simulink model "et_robocon_dev_guy3"  (R2013b)
settings: Solver=FixedStepDiscrete  SolverMode=SingleTasking  StartTime=0.0  StopTime=inf  FixedStep=balancer_ts  RelTol=1e-3
undefined symbols (not defined in the file): a_d, a_r, balancerStates_Bus0, Batt, battery_gain, battery_offset, cmd_max, current_mode_status, current_task_operation_status, DiscIntNeverNeededParam, exec_period, gcbh, Init_Bus0, K, k_f, k_i, k_phidot, k_thetadot, lightCalib, R, realtime, STATE, TRACK_MODE_LIST, ts2, W
libraries: legonxtlib x34, simulink x11, simulink_extras x4
(part 1 of 4)
settings Model: DataDictionary=mainDict.sldd  ExtModeTrigDuration=2  Creator=mbiesiad  LastModifiedBy=grouleau
settings ConfigSet: Description=Use this configuration to communicate between two robots. This robot is the master.
settings OptimizationCC: OptimizeModelRefInitCode=on  LifeSpan=1
settings DebuggingCC: UnderspecifiedInitializationDetection=Simplified  SolverPrmCheckMsg=none  ParameterPrecisionLossMsg=none  SignalLabelMismatchMsg=error  NonBusSignalsTreatedAsBus=error
settings HardwareCC: ProdLargestAtomicInteger=Long  ProdLargestAtomicFloat=Float  ProdEndianess=LittleEndian  ProdHWDeviceType=ARM Compatible->ARM 7
settings RTWCC: SystemTargetFile=realtime.tlc  GenerateMakefile=off  TemplateMakefile=realtime.tmf  Description=Run on Target Hardware  RTWVerbose=off  ProcessScript=realtime_make_rtw_hook
settings STFCustomTargetCC: TargetLibSuffix=.a  GenerateSampleERTMain=on  ERTCustomFileBanners=on  SupportNonInlinedSFcns=off  SupportVariableSizeSignals=on  MATLABClassNameForMDSCustomization=Simulink.SoftwareTarget.ERTCustomization  GRTInterface=off  SystemTargetFile=realtime.tlc
settings ERTTargetCC: CodeReplacementLibrary=ANSI_C  GenerateSampleERTMain=on  ParMdlRefBuildCompliant=off  CompOptLevelCompliant=off  ConcurrentExecutionCompliant=off  CombineOutputUpdateFcns=off  ERTFirstTimeCompliant=off  SupportContinuousTime=on  SupportVariableSizeSignals=on  ModelStepFunctionPrototypeControlCompliant=off  CPPClassGenCompliant=off  ExtModeTransport=1  ExtModeMexFile=ext_serial_win32_comm_no_acks_rtt_byteswap  ExtModeMexArgs=0 1 9600  InlinedParameterPlacement=NonHierarchical  ERTSrcFileBannerTemplate=realtime_code_template.cgt  ERTHdrFileBannerTemplate=realtime_code_template.cgt  ERTDataSrcFileTemplate=realtime_code_template.cgt  ERTDataHdrFileTemplate=realtime_code_template.cgt  ERTCustomFileTemplate=realtime_file_process.tlc

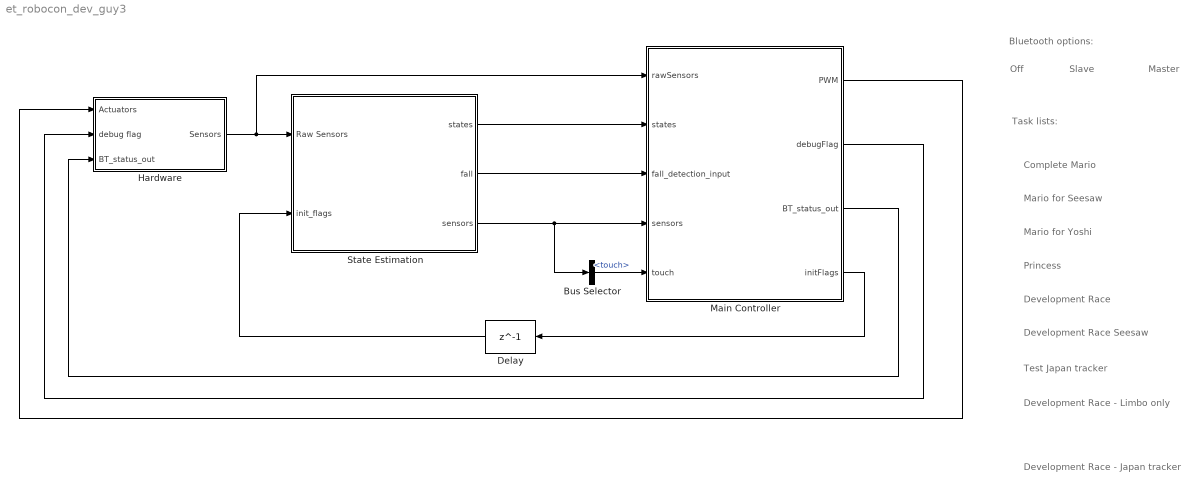
== system et_robocon_dev_guy3 ==
  note: Task lists:
  note: Bluetooth options:
  note: Slave
  note: Complete Mario
  note: Princess
  note: Mario for Seesaw
  note: Mario for Yoshi
  note: Development Race
  note: Development Race Seesaw
  note: Master
  note: Off
  note: Development Race - Japan tracker
  note: Test Japan tracker
  note: Development Race - Limbo only
  Bus Selector : BusSelector  OutputSignals=touch
  Delay : Delay  DelayLength=1
  Hardware : Subsystem  VariantControl=Variant1
  Main Controller : Stateflow chart  TreatAsAtomicUnit=on
  State Estimation : Subsystem
  wires:
  State Estimation/2(fall) -> Main Controller/3(fall_detection_input)
  State Estimation/3(sensors) -> Bus Selector/1, Main Controller/4(sensors)
  Bus Selector/1 -> Main Controller/5(touch)  "<touch>"
  Hardware/1(Sensors) -> Main Controller/1(rawSensors), State Estimation/1(Raw Sensors)
  Main Controller/4(initFlags) -> Delay/1
  State Estimation/1(states) -> Main Controller/2(states)
  Delay/1 -> State Estimation/2(init_flags)
  Main Controller/2(debugFlag) -> Hardware/2(debug flag)
  Main Controller/1(PWM) -> Hardware/1(Actuators)
  Main Controller/3(BT_status_out) -> Hardware/3(BT_status_out)

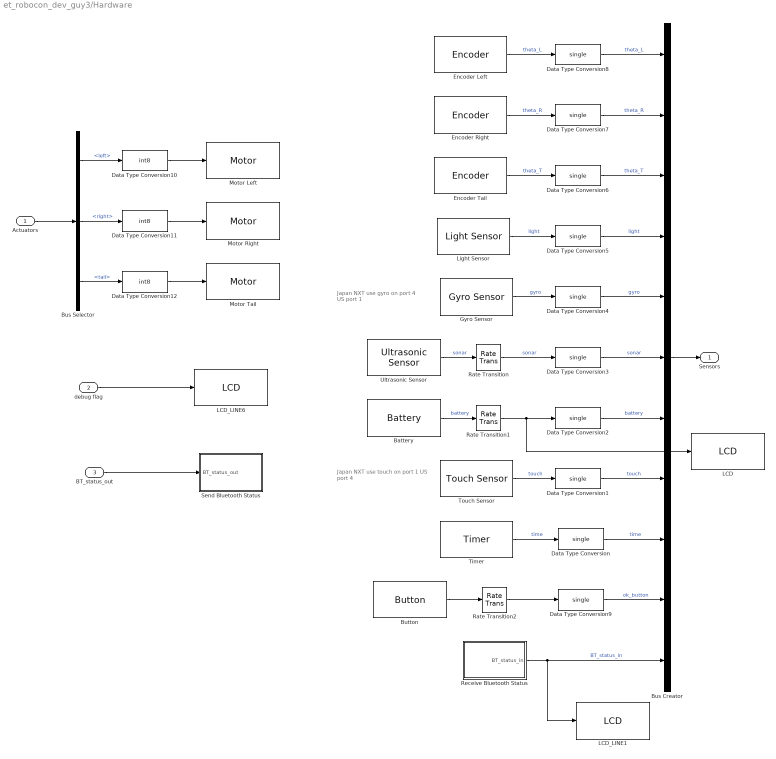
== system et_robocon_dev_guy3/Hardware ==
  note: Japan NXT use gyro on port 4
      | US port 1
  note: Japan NXT use touch  on port 1
      | US port 4
  Actuators : Inport
  debug flag : Inport  Port=2
  BT_status_out : Inport  Port=3
  Battery : legonxtlib/Battery  sampleTime=.1
  Bus Creator : BusCreator  Inputs=11
  Bus Selector : BusSelector  OutputSignals=left,right,tail
  Button : legonxtlib/Button  buttonType=Middle orange  sampleTime=0.1
  Data Type Conversion{,1..9} (10 alike) : DataTypeConversion  OutDataTypeStr=single
  Data Type Conversion10 : DataTypeConversion  OutDataTypeStr=int8  SaturateOnIntegerOverflow=on
  Data Type Conversion11 : DataTypeConversion  OutDataTypeStr=int8  SaturateOnIntegerOverflow=on
  Data Type Conversion12 : DataTypeConversion  OutDataTypeStr=int8  SaturateOnIntegerOverflow=on
  Encoder Left : legonxtlib/Encoder  portNumber=C  opMode=No reset  sampleTime=0.004
  Encoder Right : legonxtlib/Encoder  portNumber=B  opMode=No reset  sampleTime=0.004
  Encoder Tail : legonxtlib/Encoder  portNumber=A  opMode=No reset  sampleTime=0.004
  Gyro Sensor : legonxtlib/Gyro Sensor  portNumber=4  outputMode=Raw A/D (0 - 1023)  offset=599  sampleTime=0.004
  LCD : legonxtlib/LCD  slcdStr=Batt:  slcdLine=3  slcdFormat=Decimal
  LCD_LINE1 : legonxtlib/LCD  slcdStr=BTSTATUS  slcdLine=2  slcdFormat=Decimal
  LCD_LINE6 : legonxtlib/LCD  slcdStr=STATE:  slcdLine=1  slcdFormat=Decimal
  Light Sensor : legonxtlib/Light Sensor  portNumber=3  outputMode=Raw A/D (1023 - 0)  lightOn=on  sampleTime=0.004
  Motor Left : legonxtlib/Motor  sportNumber=C  sstopAction=Brake
  Motor Right : legonxtlib/Motor  sportNumber=B  sstopAction=Brake
  Motor Tail : legonxtlib/Motor  sportNumber=A  sstopAction=Brake
  Rate Transition : RateTransition  OutPortSampleTime=0.004
  Rate Transition1 : RateTransition  OutPortSampleTime=0.004
  Rate Transition2 : RateTransition  OutPortSampleTime=0.004
  Receive Bluetooth Status : Subsystem  Variant=on
  Send Bluetooth Status : Subsystem  Variant=on
  Timer : legonxtlib/Timer  sampleTime=0.004
  Touch Sensor : legonxtlib/Touch Sensor  portNumber=1  sampleTime=0.004
  Ultrasonic Sensor : legonxtlib/Ultrasonic Sensor  PortNumber=2  sampleTime=0.02
  Sensors : Outport
  wires:
  Receive Bluetooth Status/1(BT_status_in) -> LCD_LINE1/1, Bus Creator/11  "BT_status_in"
  debug flag/1 -> LCD_LINE6/1
  Data Type Conversion9/1 -> Bus Creator/10  "ok_button"
  Rate Transition2/1 -> Data Type Conversion9/1
  Button/1 -> Rate Transition2/1
  Rate Transition1/1 -> LCD/1, Data Type Conversion2/1
  Data Type Conversion8/1 -> Bus Creator/1  "theta_L"
  Data Type Conversion7/1 -> Bus Creator/2  "theta_R"
  Data Type Conversion6/1 -> Bus Creator/3  "theta_T"
  Data Type Conversion5/1 -> Bus Creator/4  "light"
  Data Type Conversion4/1 -> Bus Creator/5  "gyro"
  Data Type Conversion3/1 -> Bus Creator/6  "sonar"
  Data Type Conversion2/1 -> Bus Creator/7  "battery"
  Data Type Conversion1/1 -> Bus Creator/8  "touch"
  Data Type Conversion/1 -> Bus Creator/9  "time"
  Rate Transition/1 -> Data Type Conversion3/1  "sonar"
  Ultrasonic Sensor/1 -> Rate Transition/1  "sonar"
  Bus Selector/3 -> Data Type Conversion12/1  "<tail>"
  Encoder Tail/1 -> Data Type Conversion6/1  "theta_T"
  Light Sensor/1 -> Data Type Conversion5/1  "light"
  Bus Selector/2 -> Data Type Conversion11/1  "<right>"
  Bus Selector/1 -> Data Type Conversion10/1  "<left>"
  Touch Sensor/1 -> Data Type Conversion1/1  "touch"
  Bus Creator/1 -> Sensors/1
  Battery/1 -> Rate Transition1/1  "battery"
  Gyro Sensor/1 -> Data Type Conversion4/1  "gyro"
  Encoder Right/1 -> Data Type Conversion7/1  "theta_R"
  Encoder Left/1 -> Data Type Conversion8/1  "theta_L"
  Timer/1 -> Data Type Conversion/1  "time"
  Actuators/1 -> Bus Selector/1
  Data Type Conversion10/1 -> Motor Left/1
  Data Type Conversion11/1 -> Motor Right/1
  Data Type Conversion12/1 -> Motor Tail/1
  BT_status_out/1 -> Send Bluetooth Status/1(BT_status_out)

== system et_robocon_dev_guy3/Main Controller/normal_operation_modes.gyro_calibration_mode ==
  sensors : Inport
  touch : Inport  Port=2
  " Demux " : Demux  Outputs=2
  " SFunction " : S-Function  Tag=Stateflow S-Function et_robocon_dev_guy3 10  FunctionName=sf_sfun  PortCounts=[3 6]  EnableBusSupport=off
  gyro_calibration_mode.GyroCalibration.Speak : Subsystem
      settings: UndoDeleteFcn=Stateflow.SLINSF.SimulinkMan.restorePreDeleteFcn  PreDeleteFcn=Stateflow.SLINSF.SimulinkMan.removePreDeleteFcn
  gyro_calibration_mode.GyroCalibration.tail_controller : Subsystem
      settings: UndoDeleteFcn=Stateflow.SLINSF.SimulinkMan.restorePreDeleteFcn  PreDeleteFcn=Stateflow.SLINSF.SimulinkMan.removePreDeleteFcn
  debugFlag : Outport
  initFlags : Outport  Port=2
  PWM : Outport  Port=3
  wires:
  sensors/1 -> " SFunction "/1
  touch/1 -> " SFunction "/2
  " SFunction "/2 -> debugFlag/1  "debugFlag"
  " SFunction "/3 -> initFlags/1  "initFlags"
  " SFunction "/4 -> PWM/1  "PWM"
  " SFunction "/5 -> gyro_calibration_mode.GyroCalibration.tail_controller/1(current)
  " SFunction "/6 -> gyro_calibration_mode.GyroCalibration.tail_controller/2(desired)
  gyro_calibration_mode.GyroCalibration.tail_controller/1(cmd) -> " SFunction "/3
  " Demux "/1 -> gyro_calibration_mode.GyroCalibration.tail_controller/Trigger
  " Demux "/2 -> gyro_calibration_mode.GyroCalibration.Speak/Trigger
  " SFunction "/1 -> " Demux "/1

== system et_robocon_dev_guy3/Main Controller/normal_operation_modes.light_calibration_limbo ==
  sensors : Inport
  touch : Inport  Port=2
  " Demux " : Demux  Outputs=2
  " SFunction " : S-Function  Tag=Stateflow S-Function et_robocon_dev_guy3 4  FunctionName=sf_sfun  PortCounts=[3 5]  EnableBusSupport=off
  light_sensor_calibration_limbo.Speak : Subsystem
      settings: UndoDeleteFcn=Stateflow.SLINSF.SimulinkMan.restorePreDeleteFcn  PreDeleteFcn=Stateflow.SLINSF.SimulinkMan.removePreDeleteFcn
  light_sensor_calibration_limbo.tail_controller : Subsystem
      settings: UndoDeleteFcn=Stateflow.SLINSF.SimulinkMan.restorePreDeleteFcn  PreDeleteFcn=Stateflow.SLINSF.SimulinkMan.removePreDeleteFcn
  debugFlag : Outport
  PWM : Outport  Port=2
  wires:
  sensors/1 -> " SFunction "/1
  touch/1 -> " SFunction "/2
  " SFunction "/2 -> debugFlag/1  "debugFlag"
  " SFunction "/3 -> PWM/1  "PWM"
  " SFunction "/4 -> light_sensor_calibration_limbo.tail_controller/1(current)
  " SFunction "/5 -> light_sensor_calibration_limbo.tail_controller/2(desired)
  light_sensor_calibration_limbo.tail_controller/1(cmd) -> " SFunction "/3
  " Demux "/1 -> light_sensor_calibration_limbo.tail_controller/Trigger
  " Demux "/2 -> light_sensor_calibration_limbo.Speak/Trigger
  " SFunction "/1 -> " Demux "/1

== system et_robocon_dev_guy3/Main Controller/normal_operation_modes.light_calibration_on_tail ==
  sensors : Inport
  touch : Inport  Port=2
  " Demux " : Demux  Outputs=2
  " SFunction " : S-Function  Tag=Stateflow S-Function et_robocon_dev_guy3 9  FunctionName=sf_sfun  PortCounts=[3 5]  EnableBusSupport=off
  light_sensor_calibration_oon_tail.Speak : Subsystem
      settings: UndoDeleteFcn=Stateflow.SLINSF.SimulinkMan.restorePreDeleteFcn  PreDeleteFcn=Stateflow.SLINSF.SimulinkMan.removePreDeleteFcn
  light_sensor_calibration_oon_tail.tail_controller : Subsystem
      settings: UndoDeleteFcn=Stateflow.SLINSF.SimulinkMan.restorePreDeleteFcn  PreDeleteFcn=Stateflow.SLINSF.SimulinkMan.removePreDeleteFcn
  debugFlag : Outport
  PWM : Outport  Port=2
  wires:
  sensors/1 -> " SFunction "/1
  touch/1 -> " SFunction "/2
  " SFunction "/2 -> debugFlag/1  "debugFlag"
  " SFunction "/3 -> PWM/1  "PWM"
  " SFunction "/4 -> light_sensor_calibration_oon_tail.tail_controller/1(current)
  " SFunction "/5 -> light_sensor_calibration_oon_tail.tail_controller/2(desired)
  light_sensor_calibration_oon_tail.tail_controller/1(cmd) -> " SFunction "/3
  " Demux "/1 -> light_sensor_calibration_oon_tail.tail_controller/Trigger
  " Demux "/2 -> light_sensor_calibration_oon_tail.Speak/Trigger
  " SFunction "/1 -> " Demux "/1

== system et_robocon_dev_guy3/Main Controller/normal_operation_modes.light_calibration_up ==
  sensors : Inport
  touch : Inport  Port=2
  " Demux " : Demux
  " SFunction " : S-Function  Tag=Stateflow S-Function et_robocon_dev_guy3 8  FunctionName=sf_sfun  PortCounts=[4 7]  EnableBusSupport=off
  Speak : Subsystem
      settings: UndoDeleteFcn=Stateflow.SLINSF.SimulinkMan.restorePreDeleteFcn  PreDeleteFcn=Stateflow.SLINSF.SimulinkMan.removePreDeleteFcn
  light_sensor_calibration_up.processLight : Subsystem
      settings: UndoDeleteFcn=Stateflow.SLINSF.SimulinkMan.restorePreDeleteFcn  PreDeleteFcn=Stateflow.SLINSF.SimulinkMan.removePreDeleteFcn
  light_sensor_calibration_up.tail_controller : Subsystem
      settings: UndoDeleteFcn=Stateflow.SLINSF.SimulinkMan.restorePreDeleteFcn  PreDeleteFcn=Stateflow.SLINSF.SimulinkMan.removePreDeleteFcn
  light_sensor_calibration_up.turnLightOn : Subsystem
      settings: UndoDeleteFcn=Stateflow.SLINSF.SimulinkMan.restorePreDeleteFcn  PreDeleteFcn=Stateflow.SLINSF.SimulinkMan.removePreDeleteFcn
  debugFlag : Outport
  PWM : Outport  Port=2
  initFlags : Outport  Port=3
  wires:
  sensors/1 -> " SFunction "/1
  touch/1 -> " SFunction "/2
  " SFunction "/2 -> debugFlag/1  "debugFlag"
  " SFunction "/3 -> PWM/1  "PWM"
  " SFunction "/4 -> initFlags/1  "initFlags"
  " Demux "/1 -> Speak/Trigger
  " SFunction "/5 -> light_sensor_calibration_up.tail_controller/1(current)
  " SFunction "/6 -> light_sensor_calibration_up.tail_controller/2(desired)
  light_sensor_calibration_up.tail_controller/1(cmd) -> " SFunction "/3
  " Demux "/2 -> light_sensor_calibration_up.tail_controller/Trigger
  " SFunction "/7 -> light_sensor_calibration_up.processLight/1(rawLight)
  light_sensor_calibration_up.processLight/1(filteredLight) -> " SFunction "/4
  " Demux "/3 -> light_sensor_calibration_up.processLight/Trigger
  " Demux "/4 -> light_sensor_calibration_up.turnLightOn/Trigger
  " SFunction "/1 -> " Demux "/1

== system et_robocon_dev_guy3/Main Controller/normal_operation_modes.limbo_mode ==
  sensors : Inport
  states : Inport  Port=2
  " Demux " : Demux  Outputs=3
  " SFunction " : S-Function  Tag=Stateflow S-Function et_robocon_dev_guy3 6  FunctionName=sf_sfun  PortCounts=[5 11]  EnableBusSupport=off
  Speak : Subsystem
      settings: UndoDeleteFcn=Stateflow.SLINSF.SimulinkMan.restorePreDeleteFcn  PreDeleteFcn=Stateflow.SLINSF.SimulinkMan.removePreDeleteFcn
  lineTrackLimbo : Subsystem
      settings: UndoDeleteFcn=Stateflow.SLINSF.SimulinkMan.restorePreDeleteFcn  PreDeleteFcn=Stateflow.SLINSF.SimulinkMan.removePreDeleteFcn
  tail_controller : Subsystem
      settings: UndoDeleteFcn=Stateflow.SLINSF.SimulinkMan.restorePreDeleteFcn  PreDeleteFcn=Stateflow.SLINSF.SimulinkMan.removePreDeleteFcn
  PWM : Outport
  debugFlag : Outport  Port=2
  wires:
  sensors/1 -> " SFunction "/1
  states/1 -> " SFunction "/2
  " SFunction "/2 -> PWM/1  "PWM"
  " SFunction "/3 -> debugFlag/1  "debugFlag"
  " SFunction "/4 -> tail_controller/1(current)
  " SFunction "/5 -> tail_controller/2(desired)
  tail_controller/1(cmd) -> " SFunction "/3
  " Demux "/1 -> tail_controller/Trigger
  " SFunction "/6 -> lineTrackLimbo/1(sensors)
  " SFunction "/7 -> lineTrackLimbo/2(lightCalib)
  " SFunction "/8 -> lineTrackLimbo/3(forwardSpeed)
  " SFunction "/9 -> lineTrackLimbo/4(desLight)
  " SFunction "/10 -> lineTrackLimbo/5(raceLight)
  " SFunction "/11 -> lineTrackLimbo/6(wheelControl)
  lineTrackLimbo/1(PWM_left) -> " SFunction "/4
  lineTrackLimbo/2(PWM_right) -> " SFunction "/5
  " Demux "/2 -> lineTrackLimbo/Trigger
  " Demux "/3 -> Speak/Trigger
  " SFunction "/1 -> " Demux "/1

== system et_robocon_dev_guy3/Main Controller/normal_operation_modes.line_tracking_mode ==
  sensors : Inport
  touch : Inport  Port=2
  rawSensors : Inport  Port=3
  " Demux " : Demux  Outputs=7
  " SFunction " : S-Function  Tag=Stateflow S-Function et_robocon_dev_guy3 2  FunctionName=sf_sfun  PortCounts=[12 16]  EnableBusSupport=off
  line_tracking_mode.Speak : Subsystem
      settings: UndoDeleteFcn=Stateflow.SLINSF.SimulinkMan.restorePreDeleteFcn  PreDeleteFcn=Stateflow.SLINSF.SimulinkMan.removePreDeleteFcn
  line_tracking_mode.Track.analyzeEncoders : Subsystem
      settings: UndoDeleteFcn=Stateflow.SLINSF.SimulinkMan.restorePreDeleteFcn  PreDeleteFcn=Stateflow.SLINSF.SimulinkMan.removePreDeleteFcn
  line_tracking_mode.Track.lineTracker : Subsystem
      settings: UndoDeleteFcn=Stateflow.SLINSF.SimulinkMan.restorePreDeleteFcn  PreDeleteFcn=Stateflow.SLINSF.SimulinkMan.removePreDeleteFcn
  line_tracking_mode.Track.processLight : Subsystem
      settings: UndoDeleteFcn=Stateflow.SLINSF.SimulinkMan.restorePreDeleteFcn  PreDeleteFcn=Stateflow.SLINSF.SimulinkMan.removePreDeleteFcn
  line_tracking_mode.balanceControl : Subsystem
      settings: UndoDeleteFcn=Stateflow.SLINSF.SimulinkMan.restorePreDeleteFcn  PreDeleteFcn=Stateflow.SLINSF.SimulinkMan.removePreDeleteFcn
  line_tracking_mode.tail_controller : Subsystem
      settings: UndoDeleteFcn=Stateflow.SLINSF.SimulinkMan.restorePreDeleteFcn  PreDeleteFcn=Stateflow.SLINSF.SimulinkMan.removePreDeleteFcn
  line_tracking_mode.turnLightOn : Subsystem
      settings: UndoDeleteFcn=Stateflow.SLINSF.SimulinkMan.restorePreDeleteFcn  PreDeleteFcn=Stateflow.SLINSF.SimulinkMan.removePreDeleteFcn
  PWM : Outport
  debugFlag : Outport  Port=2
  wires:
  sensors/1 -> " SFunction "/1
  touch/1 -> " SFunction "/2
  rawSensors/1 -> " SFunction "/3
  " SFunction "/2 -> PWM/1  "PWM"
  " SFunction "/3 -> debugFlag/1  "debugFlag"
  " SFunction "/4 -> line_tracking_mode.Track.processLight/1(rawLight)
  " SFunction "/5 -> line_tracking_mode.Track.processLight/2(bias)
  " SFunction "/6 -> line_tracking_mode.Track.processLight/3(lightCalib)
  line_tracking_mode.Track.processLight/1(normalizedLight) -> " SFunction "/4
  line_tracking_mode.Track.processLight/2(filteredLight) -> " SFunction "/5
  " Demux "/1 -> line_tracking_mode.Track.processLight/Trigger
  " SFunction "/7 -> line_tracking_mode.Track.analyzeEncoders/1(rawSensors)
  line_tracking_mode.Track.analyzeEncoders/1(AngleCount) -> " SFunction "/6
  line_tracking_mode.Track.analyzeEncoders/2(EncoderReset) -> " SFunction "/7
  line_tracking_mode.Track.analyzeEncoders/3(Angle) -> " SFunction "/8
  " Demux "/2 -> line_tracking_mode.Track.analyzeEncoders/Trigger
  " SFunction "/8 -> line_tracking_mode.Track.lineTracker/1(lightSignal)
  " SFunction "/9 -> line_tracking_mode.Track.lineTracker/2(flagSteering)
  " SFunction "/10 -> line_tracking_mode.Track.lineTracker/3(PID)
  " SFunction "/11 -> line_tracking_mode.Track.lineTracker/4(fwd)
  line_tracking_mode.Track.lineTracker/1(cmd) -> " SFunction "/9
  " Demux "/3 -> line_tracking_mode.Track.lineTracker/Trigger
  " SFunction "/12 -> line_tracking_mode.balanceControl/1(rawSensors)
  " SFunction "/13 -> line_tracking_mode.balanceControl/2(lineTrackCmd)
  " SFunction "/14 -> line_tracking_mode.balanceControl/3(gyroTrick)
  line_tracking_mode.balanceControl/1(leftPWM) -> " SFunction "/10
  line_tracking_mode.balanceControl/2(rightPWM) -> " SFunction "/11
  " Demux "/4 -> line_tracking_mode.balanceControl/Trigger
  " SFunction "/15 -> line_tracking_mode.tail_controller/1(current)
  " SFunction "/16 -> line_tracking_mode.tail_controller/2(desired)
  line_tracking_mode.tail_controller/1(cmd) -> " SFunction "/12
  " Demux "/5 -> line_tracking_mode.tail_controller/Trigger
  " Demux "/6 -> line_tracking_mode.turnLightOn/Trigger
  " Demux "/7 -> line_tracking_mode.Speak/Trigger
  " SFunction "/1 -> " Demux "/1

== system et_robocon_dev_guy3/Main Controller/normal_operation_modes.see_saw ==
  states : Inport
  sensors : Inport  Port=2
  " Demux " : Demux  Outputs=7
  " SFunction " : S-Function  Tag=Stateflow S-Function et_robocon_dev_guy3 7  FunctionName=sf_sfun  Parameters=balancerStates_Bus0  PortCounts=[7 21]  EnableBusSupport=off
  see_saw_mode.DispTheta : Subsystem
      settings: UndoDeleteFcn=Stateflow.SLINSF.SimulinkMan.restorePreDeleteFcn  PreDeleteFcn=Stateflow.SLINSF.SimulinkMan.removePreDeleteFcn
  see_saw_mode.Speak : Subsystem
      settings: UndoDeleteFcn=Stateflow.SLINSF.SimulinkMan.restorePreDeleteFcn  PreDeleteFcn=Stateflow.SLINSF.SimulinkMan.removePreDeleteFcn
  see_saw_mode.balance_ctrl : Subsystem
      settings: UndoDeleteFcn=Stateflow.SLINSF.SimulinkMan.restorePreDeleteFcn  PreDeleteFcn=Stateflow.SLINSF.SimulinkMan.removePreDeleteFcn
  see_saw_mode.lineTracker : Subsystem
      settings: UndoDeleteFcn=Stateflow.SLINSF.SimulinkMan.restorePreDeleteFcn  PreDeleteFcn=Stateflow.SLINSF.SimulinkMan.removePreDeleteFcn
  see_saw_mode.phiController : Subsystem
      settings: UndoDeleteFcn=Stateflow.SLINSF.SimulinkMan.restorePreDeleteFcn  PreDeleteFcn=Stateflow.SLINSF.SimulinkMan.removePreDeleteFcn
  see_saw_mode.processLight : Subsystem
      settings: UndoDeleteFcn=Stateflow.SLINSF.SimulinkMan.restorePreDeleteFcn  PreDeleteFcn=Stateflow.SLINSF.SimulinkMan.removePreDeleteFcn
  see_saw_mode.tail_controller : Subsystem
      settings: UndoDeleteFcn=Stateflow.SLINSF.SimulinkMan.restorePreDeleteFcn  PreDeleteFcn=Stateflow.SLINSF.SimulinkMan.removePreDeleteFcn
  PWM : Outport
  initFlags : Outport  Port=2
  debugFlag : Outport  Port=3
  wires:
  states/1 -> " SFunction "/1
  sensors/1 -> " SFunction "/2
  " SFunction "/2 -> PWM/1  "PWM"
  " SFunction "/3 -> initFlags/1  "initFlags"
  " SFunction "/4 -> debugFlag/1  "debugFlag"
  " SFunction "/5 -> see_saw_mode.processLight/1(rawLight)
  " SFunction "/6 -> see_saw_mode.processLight/2(lightCalib)
  see_saw_mode.processLight/1(light) -> " SFunction "/3
  " Demux "/1 -> see_saw_mode.processLight/Trigger
  " SFunction "/7 -> see_saw_mode.DispTheta/1(light)
  " SFunction "/8 -> see_saw_mode.DispTheta/2(turningPWM)
  " Demux "/2 -> see_saw_mode.DispTheta/Trigger
  " SFunction "/9 -> see_saw_mode.phiController/1(phi)
  " SFunction "/10 -> see_saw_mode.phiController/2(desiredPhi)
  " SFunction "/11 -> see_saw_mode.phiController/3(battery)
  see_saw_mode.phiController/1(cmd) -> " SFunction "/4
  " Demux "/3 -> see_saw_mode.phiController/Trigger
  " SFunction "/12 -> see_saw_mode.lineTracker/1(desiredLight)
  " SFunction "/13 -> see_saw_mode.lineTracker/2(light)
  " SFunction "/14 -> see_saw_mode.lineTracker/3(trackingPower)
  " SFunction "/15 -> see_saw_mode.lineTracker/4(battery)
  see_saw_mode.lineTracker/1(cmd) -> " SFunction "/5
  " Demux "/4 -> see_saw_mode.lineTracker/Trigger
  " Demux "/5 -> see_saw_mode.Speak/Trigger
  " SFunction "/16 -> see_saw_mode.tail_controller/1(current)
  " SFunction "/17 -> see_saw_mode.tail_controller/2(desired)
  see_saw_mode.tail_controller/1(cmd) -> " SFunction "/6
  " Demux "/6 -> see_saw_mode.tail_controller/Trigger
  " SFunction "/18 -> see_saw_mode.balance_ctrl/1(balancerStates)
  " SFunction "/19 -> see_saw_mode.balance_ctrl/2(desired_velocity)
  " SFunction "/20 -> see_saw_mode.balance_ctrl/3(battery)
  " SFunction "/21 -> see_saw_mode.balance_ctrl/4(desired_psi)
  see_saw_mode.balance_ctrl/1(cmd) -> " SFunction "/7
  " Demux "/7 -> see_saw_mode.balance_ctrl/Trigger
  " SFunction "/1 -> " Demux "/1

== system et_robocon_dev_guy3/State Estimation ==
  Raw Sensors : Inport
  init_flags : Inport  Port=2
  Bus Selector1 : BusSelector  OutputSignals=tail,gyroInit,gyroReset,theta,fall
  Data Type Conversion Unit Conversion Tail Initialization : Subsystem
  Fall Detection : Subsystem
  Gyro Processing : Subsystem
  StateEstimation : Subsystem
  states : Outport
  fall : Outport  Port=2
  sensors : Outport  Port=3
  wires:
  Bus Selector1/3 -> Gyro Processing/3(gyroReset)  "<gyroReset>"
  Bus Selector1/4 -> StateEstimation/4(init theta)  "<theta>"
  Bus Selector1/1 -> Data Type Conversion Unit Conversion Tail Initialization/2(init_tail)  "<tail>"
  Bus Selector1/2 -> Gyro Processing/2(gyroInit)  "<gyroInit>"
  init_flags/1 -> Bus Selector1/1
  StateEstimation/1(states) -> states/1  "states"
  Data Type Conversion Unit Conversion Tail Initialization/1(y) -> Gyro Processing/1(sensors), sensors/1, StateEstimation/1(Sensors)
  Raw Sensors/1 -> Data Type Conversion Unit Conversion Tail Initialization/1(u)
  Gyro Processing/1(psi) -> StateEstimation/2(psi)
  Gyro Processing/2(psi_dot) -> StateEstimation/3(psi_dot)
  Gyro Processing/3(psi filtered) -> Fall Detection/1(gyro)
  Bus Selector1/5 -> Fall Detection/2(reset)  "<fall>"
  Fall Detection/1(fall_detected) -> fall/1

== system et_robocon_dev_guy3/Hardware/Receive Bluetooth Status ==
  note: 1) Only subsystems can be added as variant choices at this level
      | 2) Blocks cannot be connected at this level as connectivity is
      | automatically determined at simulation, based on the active variant
  BlueoothDevStart : Subsystem  VariantControl=BluetoothDevStart
  BluetoothOFF : Subsystem  VariantControl=BluetoothOFF
  BluetoothONMario : Subsystem  VariantControl=BluetoothONMario
  BluetoothONPrincess : Subsystem  VariantControl=BluetoothONPrincess
  BT_status_in : Outport

== system et_robocon_dev_guy3/Hardware/Send Bluetooth Status ==
  note: 1) Only subsystems can be added as variant choices at this level
      | 2) Blocks cannot be connected at this level as connectivity is
      | automatically determined at simulation, based on the active variant
  BT_status_out : Inport
  BluetoothDevStart : Subsystem  VariantControl=BluetoothDevStart
  BluetoothOFF : Subsystem  VariantControl=BluetoothOFF
  BluetoothONMario : Subsystem  VariantControl=BluetoothONMario
  BluetoothONPrincess : Subsystem  VariantControl=BluetoothONPrincess

== system et_robocon_dev_guy3/Main Controller/normal_operation_modes.gyro_calibration_mode/gyro_calibration_mode.GyroCalibration.Speak ==
  f : TriggerPort  TriggerType=function-call
      settings: CopyFcn=Stateflow.SLINSF.SimulinkMan.removeBlockPreDeleteFcn  PreDeleteFcn=Stateflow.SLINSF.SimulinkMan.unsafePredeleteFcn
  Constant : Constant  Value=50
  Speaker : legonxtlib/Speaker  sinputMode=Volume only  sspeakerFreq=800  sspeakerVolume=50  sspeakerDuration=100
  wires:
  Constant/1 -> Speaker/1

== system et_robocon_dev_guy3/Main Controller/normal_operation_modes.gyro_calibration_mode/gyro_calibration_mode.GyroCalibration.tail_controller ==
  note: Could be improved, PI for example
  current : Inport  OutDataTypeStr=single  PortDimensions=1
  desired : Inport  Port=2  OutDataTypeStr=single  PortDimensions=1
  f : TriggerPort  TriggerType=function-call
      settings: CopyFcn=Stateflow.SLINSF.SimulinkMan.removeBlockPreDeleteFcn  PreDeleteFcn=Stateflow.SLINSF.SimulinkMan.unsafePredeleteFcn
  Gain : Gain  Gain=250
  Saturation : Saturate  UpperLimit=100  LowerLimit=-100  OutDataTypeStr=single
  Sum : Sum  Inputs=|+-
  cmd : Outport  OutDataTypeStr=single  PortDimensions=1  InitialOutput=0
  wires:
  Saturation/1 -> cmd/1
  Gain/1 -> Saturation/1
  desired/1 -> Sum/1
  current/1 -> Sum/2
  Sum/1 -> Gain/1

== system et_robocon_dev_guy3/Main Controller/normal_operation_modes.light_calibration_limbo/light_sensor_calibration_limbo.Speak ==
  f : TriggerPort  TriggerType=function-call
      settings: CopyFcn=Stateflow.SLINSF.SimulinkMan.removeBlockPreDeleteFcn  PreDeleteFcn=Stateflow.SLINSF.SimulinkMan.unsafePredeleteFcn
  Constant : Constant  Value=50
  Speaker : legonxtlib/Speaker  sinputMode=Volume only  sspeakerFreq=800  sspeakerVolume=50  sspeakerDuration=100
  wires:
  Constant/1 -> Speaker/1

== system et_robocon_dev_guy3/Main Controller/normal_operation_modes.light_calibration_limbo/light_sensor_calibration_limbo.tail_controller ==
  note: Could be improved, PI for example
  current : Inport  OutDataTypeStr=single  PortDimensions=1
  desired : Inport  Port=2  OutDataTypeStr=single  PortDimensions=1
  f : TriggerPort  TriggerType=function-call
      settings: CopyFcn=Stateflow.SLINSF.SimulinkMan.removeBlockPreDeleteFcn  PreDeleteFcn=Stateflow.SLINSF.SimulinkMan.unsafePredeleteFcn
  Gain : Gain  Gain=250
  Saturation : Saturate  UpperLimit=100  LowerLimit=-100  OutDataTypeStr=single
  Sum : Sum  Inputs=|+-
  cmd : Outport  OutDataTypeStr=single  PortDimensions=1  InitialOutput=0
  wires:
  Sum/1 -> Gain/1
  current/1 -> Sum/2
  desired/1 -> Sum/1
  Gain/1 -> Saturation/1
  Saturation/1 -> cmd/1

== system et_robocon_dev_guy3/Main Controller/normal_operation_modes.light_calibration_on_tail/light_sensor_calibration_oon_tail.Speak ==
  f : TriggerPort  TriggerType=function-call
      settings: CopyFcn=Stateflow.SLINSF.SimulinkMan.removeBlockPreDeleteFcn  PreDeleteFcn=Stateflow.SLINSF.SimulinkMan.unsafePredeleteFcn
  Constant : Constant  Value=50
  Speaker : legonxtlib/Speaker  sinputMode=Volume only  sspeakerFreq=800  sspeakerVolume=50  sspeakerDuration=100
  wires:
  Constant/1 -> Speaker/1

== system et_robocon_dev_guy3/Main Controller/normal_operation_modes.light_calibration_on_tail/light_sensor_calibration_oon_tail.tail_controller ==
  note: Could be improved, PI for example
  current : Inport  OutDataTypeStr=single  PortDimensions=1
  desired : Inport  Port=2  OutDataTypeStr=single  PortDimensions=1
  f : TriggerPort  TriggerType=function-call
      settings: CopyFcn=Stateflow.SLINSF.SimulinkMan.removeBlockPreDeleteFcn  PreDeleteFcn=Stateflow.SLINSF.SimulinkMan.unsafePredeleteFcn
  Gain : Gain  Gain=250
  Saturation : Saturate  UpperLimit=100  LowerLimit=-100  OutDataTypeStr=single
  Sum : Sum  Inputs=|+-
  cmd : Outport  OutDataTypeStr=single  PortDimensions=1  InitialOutput=0
  wires:
  Saturation/1 -> cmd/1
  Gain/1 -> Saturation/1
  desired/1 -> Sum/1
  current/1 -> Sum/2
  Sum/1 -> Gain/1

== system et_robocon_dev_guy3/Main Controller/normal_operation_modes.light_calibration_up/Speak ==
  f : TriggerPort  TriggerType=function-call
      settings: CopyFcn=Stateflow.SLINSF.SimulinkMan.removeBlockPreDeleteFcn  PreDeleteFcn=Stateflow.SLINSF.SimulinkMan.unsafePredeleteFcn
  Constant : Constant  Value=50
  Speaker : legonxtlib/Speaker  sinputMode=Volume only  sspeakerFreq=800  sspeakerVolume=50  sspeakerDuration=100
  wires:
  Constant/1 -> Speaker/1

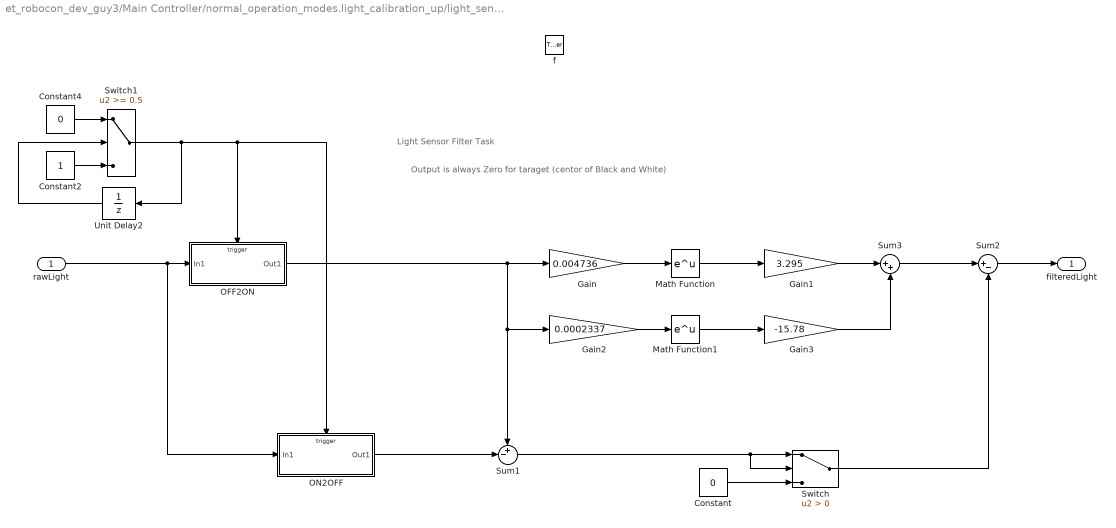
== system et_robocon_dev_guy3/Main Controller/normal_operation_modes.light_calibration_up/light_sensor_calibration_up.processLight ==
  note: Output is always Zero for taraget (centor of Black and White)
  note: Light Sensor Filter Task
  rawLight : Inport  OutDataTypeStr=single  PortDimensions=1
  f : TriggerPort  TriggerType=function-call
      settings: CopyFcn=Stateflow.SLINSF.SimulinkMan.removeBlockPreDeleteFcn  PreDeleteFcn=Stateflow.SLINSF.SimulinkMan.unsafePredeleteFcn
  Constant : Constant  Value=0  OutDataTypeStr=single  SampleTime=-1
  Constant2 : Constant  OutDataTypeStr=uint8
  Constant4 : Constant  Value=0  OutDataTypeStr=uint8
  Gain : Gain  Gain=0.004736
  Gain1 : Gain  Gain=3.295
  Gain2 : Gain  Gain=0.0002337
  Gain3 : Gain  Gain=-15.78
  Math Function : Math  SaturateOnIntegerOverflow=on
  Math Function1 : Math  SaturateOnIntegerOverflow=on
  OFF2ON : Subsystem  TreatAsAtomicUnit=on
  ON2OFF : Subsystem  TreatAsAtomicUnit=on
  Sum1 : Sum  Inputs=+-|
  Sum2 : Sum  Inputs=|+-
  Sum3 : Sum  Inputs=|++
  Switch : Switch  Criteria=u2 > Threshold  RndMeth=Simplest
  Switch1 : Switch  Threshold=0.5
  Unit Delay2 : UnitDelay  SampleTime=-1
  filteredLight : Outport  OutDataTypeStr=single  PortDimensions=1  InitialOutput=0
  wires:
  Sum2/1 -> filteredLight/1
  Switch/1 -> Sum2/2
  Sum3/1 -> Sum2/1
  Gain3/1 -> Sum3/2
  Gain1/1 -> Sum3/1
  Math Function1/1 -> Gain3/1
  Gain2/1 -> Math Function1/1
  Sum1/1 -> Switch/2, Switch/1
  Constant/1 -> Switch/3
  Math Function/1 -> Gain1/1
  Gain/1 -> Math Function/1
  OFF2ON/1(Out1) -> Gain2/1, Sum1/1, Gain/1
  ON2OFF/1(Out1) -> Sum1/2
  Unit Delay2/1 -> Switch1/2
  Constant4/1 -> Switch1/1
  Constant2/1 -> Switch1/3
  Switch1/1 -> Unit Delay2/1, OFF2ON/Trigger, ON2OFF/Trigger
  rawLight/1 -> ON2OFF/1(In1), OFF2ON/1(In1)

== system et_robocon_dev_guy3/Main Controller/normal_operation_modes.light_calibration_up/light_sensor_calibration_up.tail_controller ==
  note: Could be improved, PI for example
  current : Inport  OutDataTypeStr=single  PortDimensions=1
  desired : Inport  Port=2  OutDataTypeStr=single  PortDimensions=1
  f : TriggerPort  TriggerType=function-call
      settings: CopyFcn=Stateflow.SLINSF.SimulinkMan.removeBlockPreDeleteFcn  PreDeleteFcn=Stateflow.SLINSF.SimulinkMan.unsafePredeleteFcn
  Gain : Gain  Gain=250
  Saturation : Saturate  UpperLimit=100  LowerLimit=-100  OutDataTypeStr=single
  Sum : Sum  Inputs=|+-
  cmd : Outport  OutDataTypeStr=single  PortDimensions=1  InitialOutput=0
  wires:
  Sum/1 -> Gain/1
  current/1 -> Sum/2
  desired/1 -> Sum/1
  Gain/1 -> Saturation/1
  Saturation/1 -> cmd/1

== system et_robocon_dev_guy3/Main Controller/normal_operation_modes.light_calibration_up/light_sensor_calibration_up.turnLightOn ==
  f : TriggerPort  TriggerType=function-call
      settings: CopyFcn=Stateflow.SLINSF.SimulinkMan.removeBlockPreDeleteFcn  PreDeleteFcn=Stateflow.SLINSF.SimulinkMan.unsafePredeleteFcn
  Light Sensor Switch ON : S-Function  FunctionName=sfun_light_sw  Parameters=-1,ip,sw  EnableBusSupport=off  mask(Light Sensor ON/OFF Switch){ip=S3, sw=ON}
      mask prompts: ip "port:"; sw "switch"
      mask help: LEGO Mindstorms NXT Light Sensor switch.
      mask init:
      | [data, map]=imread('LIGHT_SENSOR.gif');
      | pic=ind2rgb(data,map);
      mask TypeOptions ip: S1 | S2 | S3 | S4
      mask TypeOptions sw: ON | OFF
      mask Display:
      | image(pic)
      | color('red')
      | fprintf('%s, %s',ip,sw)

== system et_robocon_dev_guy3/Main Controller/normal_operation_modes.limbo_mode/Speak ==
  f : TriggerPort  TriggerType=function-call
      settings: CopyFcn=Stateflow.SLINSF.SimulinkMan.removeBlockPreDeleteFcn  PreDeleteFcn=Stateflow.SLINSF.SimulinkMan.unsafePredeleteFcn
  Constant : Constant  Value=50
  Speaker : legonxtlib/Speaker  sinputMode=Volume only  sspeakerFreq=800  sspeakerVolume=50  sspeakerDuration=100
  wires:
  Constant/1 -> Speaker/1

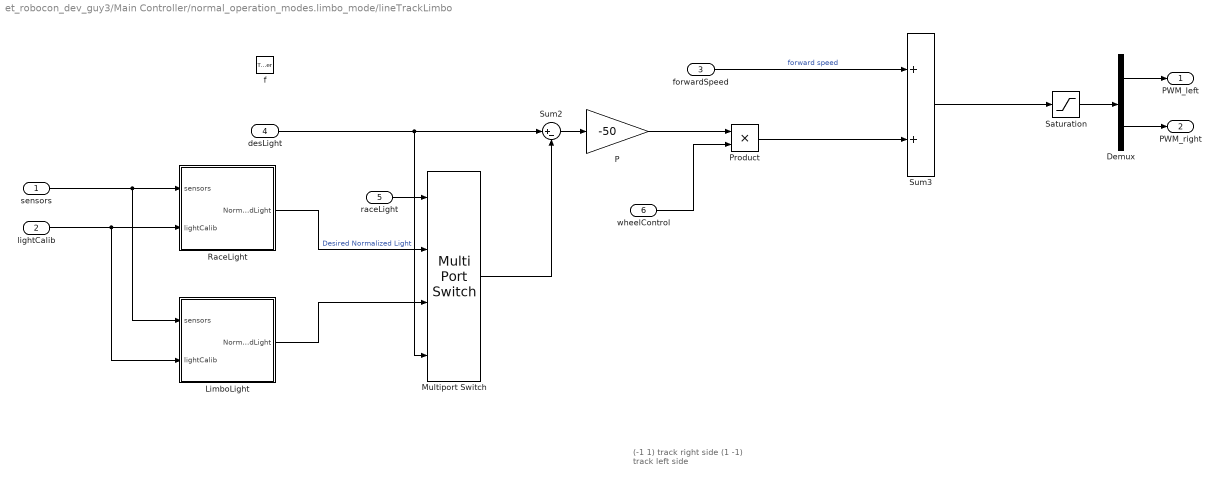
== system et_robocon_dev_guy3/Main Controller/normal_operation_modes.limbo_mode/lineTrackLimbo ==
  note: (-1 1)  track right side
      | (1 -1)  track left side
  sensors : Inport  OutDataTypeStr=Bus: Sensors_Bus  PortDimensions=1  LockScale=on
  lightCalib : Inport  Port=2  OutDataTypeStr=Bus: Light_Bus  PortDimensions=1
  forwardSpeed : Inport  Port=3  OutDataTypeStr=single  PortDimensions=[1 2]
  desLight : Inport  Port=4  OutDataTypeStr=single  PortDimensions=1
  raceLight : Inport  Port=5  OutDataTypeStr=single  PortDimensions=1
  wheelControl : Inport  Port=6  OutDataTypeStr=single  PortDimensions=[1 2]
  f : TriggerPort  TriggerType=function-call
      settings: CopyFcn=Stateflow.SLINSF.SimulinkMan.removeBlockPreDeleteFcn  PreDeleteFcn=Stateflow.SLINSF.SimulinkMan.unsafePredeleteFcn
  Demux : Demux  Outputs=2
  LimboLight : Subsystem
  Multiport Switch : MultiPortSwitch
  P : Gain  Gain=-50
  Product : Product
  RaceLight : Subsystem
  Saturation : Saturate  UpperLimit=100  LowerLimit=-100  OutDataTypeStr=single
  Sum2 : Sum  Inputs=|+-
  Sum3 : Sum
  PWM_left : Outport  OutDataTypeStr=single  PortDimensions=1
  PWM_right : Outport  Port=2  OutDataTypeStr=single  PortDimensions=1
  wires:
  Product/1 -> Sum3/2
  Sum3/1 -> Saturation/1
  wheelControl/1 -> Product/2
  Multiport Switch/1 -> Sum2/2
  RaceLight/1(NormalizedLight) -> Multiport Switch/2
  raceLight/1 -> Multiport Switch/1
  LimboLight/1(NormalizedLight) -> Multiport Switch/3
  lightCalib/1 -> RaceLight/2(lightCalib), LimboLight/2(lightCalib)
  sensors/1 -> RaceLight/1(sensors), LimboLight/1(sensors)
  desLight/1 -> Sum2/1, Multiport Switch/4  "Desired Normalized Light"
  Sum2/1 -> P/1
  Demux/1 -> PWM_left/1
  Demux/2 -> PWM_right/1
  forwardSpeed/1 -> Sum3/1  "forward speed"
  P/1 -> Product/1
  Saturation/1 -> Demux/1

== system et_robocon_dev_guy3/Main Controller/normal_operation_modes.limbo_mode/tail_controller ==
  note: Could be improved, PI for example
  current : Inport  OutDataTypeStr=single  PortDimensions=1
  desired : Inport  Port=2  OutDataTypeStr=single  PortDimensions=1
  f : TriggerPort  TriggerType=function-call
      settings: CopyFcn=Stateflow.SLINSF.SimulinkMan.removeBlockPreDeleteFcn  PreDeleteFcn=Stateflow.SLINSF.SimulinkMan.unsafePredeleteFcn
  Gain : Gain  Gain=250
  Saturation : Saturate  UpperLimit=100  LowerLimit=-100  OutDataTypeStr=single
  Sum : Sum  Inputs=|+-
  cmd : Outport  OutDataTypeStr=single  PortDimensions=1  InitialOutput=0
  wires:
  Saturation/1 -> cmd/1
  Gain/1 -> Saturation/1
  desired/1 -> Sum/1
  current/1 -> Sum/2
  Sum/1 -> Gain/1

== system et_robocon_dev_guy3/Main Controller/normal_operation_modes.line_tracking_mode/line_tracking_mode.Speak ==
  f : TriggerPort  TriggerType=function-call
      settings: CopyFcn=Stateflow.SLINSF.SimulinkMan.removeBlockPreDeleteFcn  PreDeleteFcn=Stateflow.SLINSF.SimulinkMan.unsafePredeleteFcn
  Constant : Constant  Value=50
  Speaker : legonxtlib/Speaker  sinputMode=Volume only  sspeakerFreq=800  sspeakerVolume=50  sspeakerDuration=100
  wires:
  Constant/1 -> Speaker/1

== system et_robocon_dev_guy3/Main Controller/normal_operation_modes.line_tracking_mode/line_tracking_mode.Track.analyzeEncoders ==
  rawSensors : Inport  OutDataTypeStr=Bus: Sensors_Bus  PortDimensions=1
  f : TriggerPort  TriggerType=function-call
      settings: CopyFcn=Stateflow.SLINSF.SimulinkMan.removeBlockPreDeleteFcn  PreDeleteFcn=Stateflow.SLINSF.SimulinkMan.unsafePredeleteFcn
  AngleCounter : Subsystem
  Bus Creator : BusCreator  Inputs=2
  Bus Selector : BusSelector  OutputSignals=theta_R,theta_L
  Signal Conversion : SignalConversion
  Signal Conversion1 : SignalConversion
  AngleCount : Outport  OutDataTypeStr=uint8  PortDimensions=1  InitialOutput=0
  EncoderReset : Outport  Port=2  OutDataTypeStr=single  PortDimensions=1  InitialOutput=0
  Angle : Outport  Port=3  OutDataTypeStr=single  PortDimensions=1  InitialOutput=0
  wires:
  rawSensors/1 -> Bus Selector/1
  Bus Creator/1 -> AngleCounter/1(EC)
  Bus Selector/1 -> Signal Conversion/1  "<theta_R>"
  Bus Selector/2 -> Signal Conversion1/1  "<theta_L>"
  Signal Conversion/1 -> Bus Creator/1  "R"
  Signal Conversion1/1 -> Bus Creator/2  "L"
  AngleCounter/1(AngleCount) -> AngleCount/1
  AngleCounter/2(EncoderReseted) -> EncoderReset/1
  AngleCounter/3(Angle) -> Angle/1

== system et_robocon_dev_guy3/Main Controller/normal_operation_modes.line_tracking_mode/line_tracking_mode.Track.lineTracker ==
  lightSignal : Inport  OutDataTypeStr=single  PortDimensions=1
  flagSteering : Inport  Port=2  OutDataTypeStr=single  PortDimensions=1
  PID : Inport  Port=3  OutDataTypeStr=single  PortDimensions=5
  fwd : Inport  Port=4  OutDataTypeStr=single  PortDimensions=1
  f : TriggerPort  TriggerType=function-call
      settings: CopyFcn=Stateflow.SLINSF.SimulinkMan.removeBlockPreDeleteFcn  PreDeleteFcn=Stateflow.SLINSF.SimulinkMan.unsafePredeleteFcn
  Handler : Subsystem
  Signal Conversion : SignalConversion
  SwitchForFreeSteering : Subsystem
  cmd : Outport  InitialOutput=[0 0]
  wires:
  Handler/1(cmd) -> Signal Conversion/1
  lightSignal/1 -> SwitchForFreeSteering/3(LightSens)
  SwitchForFreeSteering/1(Steering) -> Handler/1(steering)
  flagSteering/1 -> SwitchForFreeSteering/1(FlagSteering)
  PID/1 -> SwitchForFreeSteering/2(PID)
  fwd/1 -> Handler/2(fwd)
  Signal Conversion/1 -> cmd/1

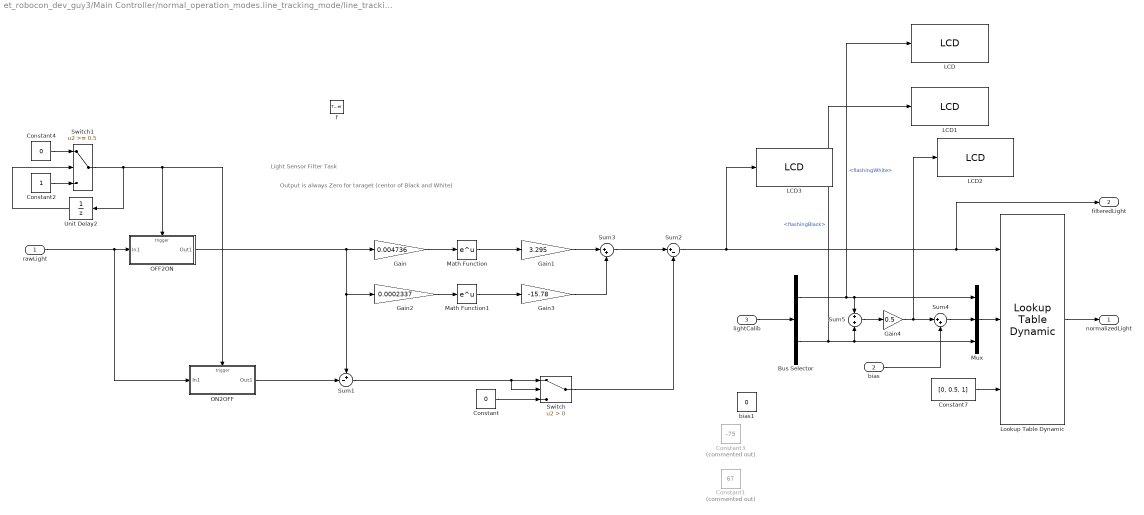
== system et_robocon_dev_guy3/Main Controller/normal_operation_modes.line_tracking_mode/line_tracking_mode.Track.processLight ==
  note: Output is always Zero for taraget (centor of Black and White)
  note: Light Sensor Filter Task
  rawLight : Inport  OutDataTypeStr=single  PortDimensions=1
  bias : Inport  Port=2  OutDataTypeStr=single  PortDimensions=1
  lightCalib : Inport  Port=3  OutDataTypeStr=Bus: Light_Bus  PortDimensions=1
  f : TriggerPort  TriggerType=function-call
      settings: CopyFcn=Stateflow.SLINSF.SimulinkMan.removeBlockPreDeleteFcn  PreDeleteFcn=Stateflow.SLINSF.SimulinkMan.unsafePredeleteFcn
  Bus Selector : BusSelector  OutputSignals=flashingWhite,flashingBlack
  Constant : Constant  Value=0  OutDataTypeStr=single  SampleTime=-1
  Constant1 : Constant  Commented=on  Value=67  OutDataTypeStr=single  SampleTime=-1
  Constant2 : Constant  OutDataTypeStr=uint8
  Constant3 : Constant  Commented=on  Value=-75  OutDataTypeStr=single  SampleTime=-1
  Constant4 : Constant  Value=0  OutDataTypeStr=uint8
  Constant7 : Constant  Value=[0, 0.5, 1]  OutDataTypeStr=single  SampleTime=-1
  Gain : Gain  Gain=0.004736
  Gain1 : Gain  Gain=3.295
  Gain2 : Gain  Gain=0.0002337
  Gain3 : Gain  Gain=-15.78
  Gain4 : Gain  Gain=0.5
  LCD : legonxtlib/LCD  slcdStr=W  slcdLine=4  slcdFormat=Decimal
  LCD1 : legonxtlib/LCD  slcdStr=B  slcdLine=5  slcdFormat=Decimal
  LCD2 : legonxtlib/LCD  slcdStr=T  slcdLine=6  slcdFormat=Decimal
  LCD3 : legonxtlib/LCD  slcdStr=L  slcdLine=7  slcdFormat=Decimal
  Lookup Table Dynamic : simulink/Lookup Tables/Lookup Table Dynamic  LookUpMeth=Interpolation-Use End Values  OutDataTypeStr=fixdt('single')  OutputDataTypeScalingMode=Specify via dialog  OutDataType=fixdt('single')  OutScaling=[]  RndMeth=Simplest  DoSatur=off
  Math Function : Math  SaturateOnIntegerOverflow=on
  Math Function1 : Math  SaturateOnIntegerOverflow=on
  Mux : Mux  Inputs=3
  OFF2ON : Subsystem  TreatAsAtomicUnit=on
  ON2OFF : Subsystem  TreatAsAtomicUnit=on
  Sum1 : Sum  Inputs=+-|
  Sum2 : Sum  Inputs=|+-
  Sum3 : Sum  Inputs=|++
  Sum4 : Sum  Inputs=|++  OutDataTypeStr=single  RndMeth=Simplest
  Sum5 : Sum  Inputs=+|+  OutDataTypeStr=single  RndMeth=Simplest
  Switch : Switch  Criteria=u2 > Threshold  RndMeth=Simplest
  Switch1 : Switch  Threshold=0.5
  Unit Delay2 : UnitDelay  SampleTime=-1
  bias1 : Constant  Value=0  OutDataTypeStr=single  SampleTime=-1
  normalizedLight : Outport  OutDataTypeStr=single  PortDimensions=1  InitialOutput=0
  filteredLight : Outport  Port=2  OutDataTypeStr=single  PortDimensions=1  InitialOutput=0
  wires:
  Bus Selector/1 -> LCD/1, Sum5/1, Mux/1  "<flashingWhite>"
  Bus Selector/2 -> LCD1/1, Mux/3, Sum5/2  "<flashingBlack>"
  Mux/1 -> Lookup Table Dynamic/2
  Sum4/1 -> Mux/2
  Gain4/1 -> LCD2/1, Sum4/1
  bias/1 -> Sum4/2
  Constant7/1 -> Lookup Table Dynamic/3
  Lookup Table Dynamic/1 -> normalizedLight/1
  Sum2/1 -> LCD3/1, filteredLight/1, Lookup Table Dynamic/1
  Switch/1 -> Sum2/2
  Sum3/1 -> Sum2/1
  Gain3/1 -> Sum3/2
  Gain1/1 -> Sum3/1
  Math Function1/1 -> Gain3/1
  Gain2/1 -> Math Function1/1
  Sum1/1 -> Switch/2, Switch/1
  Constant/1 -> Switch/3
  Math Function/1 -> Gain1/1
  Gain/1 -> Math Function/1
  OFF2ON/1(Out1) -> Gain2/1, Sum1/1, Gain/1
  ON2OFF/1(Out1) -> Sum1/2
  Unit Delay2/1 -> Switch1/2
  Constant4/1 -> Switch1/1
  Constant2/1 -> Switch1/3
  Switch1/1 -> Unit Delay2/1, OFF2ON/Trigger, ON2OFF/Trigger
  rawLight/1 -> ON2OFF/1(In1), OFF2ON/1(In1)
  Sum5/1 -> Gain4/1
  lightCalib/1 -> Bus Selector/1

== system et_robocon_dev_guy3/Main Controller/normal_operation_modes.line_tracking_mode/line_tracking_mode.balanceControl ==
  note: US robot uses 612
  rawSensors : Inport  OutDataTypeStr=Bus: Sensors_Bus  PortDimensions=1
  lineTrackCmd : Inport  Port=2  OutDataTypeStr=single  PortDimensions=2
  gyroTrick : Inport  Port=3  OutDataTypeStr=single  PortDimensions=1
  f : TriggerPort  TriggerType=function-call
      settings: CopyFcn=Stateflow.SLINSF.SimulinkMan.removeBlockPreDeleteFcn  PreDeleteFcn=Stateflow.SLINSF.SimulinkMan.unsafePredeleteFcn
  Bus Selector : BusSelector  OutputSignals=gyro,theta_L,theta_R,battery
  Constant3 : Constant  Value=600  OutDataTypeStr=uint16
  Data Type Conversion2 : DataTypeConversion  OutDataTypeStr=single  RndMeth=Simplest
      settings: AttributesFormatString=Round = %<RndMeth>
  Demux : Demux  Outputs=2
  ForSimulation : Subsystem  TreatAsAtomicUnit=on  RTWFcnName=balance_control  RTWFileName=balancer
      settings: RTWSystemCode=Nonreusable function  RTWFcnNameOpts=User specified  RTWFileNameOpts=User specified  FunctionWithSeparateData=on
  Low Pass Filter : Subsystem
  Sum : Sum
  leftPWM : Outport  OutDataTypeStr=single  PortDimensions=1
  rightPWM : Outport  Port=2
  wires:
  ForSimulation/1(pwm_l) -> rightPWM/1
  ForSimulation/2(pwm_r) -> leftPWM/1
  rawSensors/1 -> Bus Selector/1
  lineTrackCmd/1 -> Demux/1
  Bus Selector/2 -> ForSimulation/5(theta_m_l)  "<theta_L>"
  Bus Selector/3 -> ForSimulation/6(theta_m_r)  "<theta_R>"
  Constant3/1 -> Data Type Conversion2/1
  Data Type Conversion2/1 -> Sum/1  "gyro_offset"
  Bus Selector/1 -> ForSimulation/3(gyro)  "<gyro>"
  Bus Selector/4 -> Low Pass Filter/1(u)  "<battery>"
  Low Pass Filter/1(y) -> ForSimulation/7(battery)
  Demux/1 -> ForSimulation/1(cmd_forward)
  Demux/2 -> ForSimulation/2(cmd_turn)
  gyroTrick/1 -> Sum/2
  Sum/1 -> ForSimulation/4(gyro_offset)

== system et_robocon_dev_guy3/Main Controller/normal_operation_modes.line_tracking_mode/line_tracking_mode.tail_controller ==
  note: Could be improved, PI for example
  current : Inport  OutDataTypeStr=single  PortDimensions=1
  desired : Inport  Port=2  OutDataTypeStr=single  PortDimensions=1
  f : TriggerPort  TriggerType=function-call
      settings: CopyFcn=Stateflow.SLINSF.SimulinkMan.removeBlockPreDeleteFcn  PreDeleteFcn=Stateflow.SLINSF.SimulinkMan.unsafePredeleteFcn
  Gain : Gain  Gain=250
  Saturation : Saturate  UpperLimit=100  LowerLimit=-100  OutDataTypeStr=single
  Sum : Sum  Inputs=|+-
  cmd : Outport  OutDataTypeStr=single  PortDimensions=1  InitialOutput=0
  wires:
  Sum/1 -> Gain/1
  current/1 -> Sum/2
  desired/1 -> Sum/1
  Gain/1 -> Saturation/1
  Saturation/1 -> cmd/1

== system et_robocon_dev_guy3/Main Controller/normal_operation_modes.line_tracking_mode/line_tracking_mode.turnLightOn ==
  f : TriggerPort  TriggerType=function-call
      settings: CopyFcn=Stateflow.SLINSF.SimulinkMan.removeBlockPreDeleteFcn  PreDeleteFcn=Stateflow.SLINSF.SimulinkMan.unsafePredeleteFcn
  Light Sensor Switch ON : S-Function  FunctionName=sfun_light_sw  Parameters=-1,ip,sw  EnableBusSupport=off  mask(Light Sensor ON/OFF Switch){ip=S3, sw=ON}
      mask prompts: ip "port:"; sw "switch"
      mask help: LEGO Mindstorms NXT Light Sensor switch.
      mask init:
      | [data, map]=imread('LIGHT_SENSOR.gif');
      | pic=ind2rgb(data,map);
      mask TypeOptions ip: S1 | S2 | S3 | S4
      mask TypeOptions sw: ON | OFF
      mask Display:
      | image(pic)
      | color('red')
      | fprintf('%s, %s',ip,sw)

== system et_robocon_dev_guy3/Main Controller/normal_operation_modes.see_saw/see_saw_mode.DispTheta ==
  light : Inport  OutDataTypeStr=double  PortDimensions=1
  turningPWM : Inport  Port=2  OutDataTypeStr=double  PortDimensions=1
  f : TriggerPort  TriggerType=function-call
      settings: CopyFcn=Stateflow.SLINSF.SimulinkMan.removeBlockPreDeleteFcn  PreDeleteFcn=Stateflow.SLINSF.SimulinkMan.unsafePredeleteFcn
  Gain : Gain  Gain=100
  Gain1 : Gain  Gain=100
  LCD : legonxtlib/LCD  slcdStr=Theta  slcdLine=2  slcdFormat=Decimal
  LCD1 : Subsystem  InitFcn=realtime.validateBlock('LEGO MINDSTORMS NXT', gcbh, '')  mask(LEGO MINDSTORMS NXT LCD){slcdStr=turnPWM, slcdLine=3, slcdFormat=Decimal}
      mask prompts: slcdStr "Display label (maximum  8 characters):"; slcdLine "Display at line:"; slcdFormat "Display format:"
      mask help: Displays the numeric value from the block input port. The display truncates the input value to show only the integer portion. Use Display at line parameter to select the row. Use Display format parameter to select the format of the number: decimal or hexadecimal.
      mask init:
      | realtime.internal.nxtLcdSysCallback;
      mask Help: eval('realtime.helpView(''LEGO MINDSTORMS NXT'', ''legonxtlibnxtlcd'')')
      mask TypeOptions slcdLine: 1 | 2 | 3 | 4 | 5 | 6 | 7 | 8
      mask TypeOptions slcdFormat: Decimal | Hex
      mask Display:
      | [data, map]=imread('LCD.gif');pic=ind2rgb(data,map);image(pic,[0.32 0.25 0.35 0.55]);
      | lineText = sprintf('Line %d', slcdLine);
      | text(0.5, 0.15, lineText, 'horizontalAlignment', 'center');
      | port_label('input', 1, '');
      | color('blue');
      | text(0.65, 0.87, 'LEGO', 'horizontalAlignment', 'left');
  wires:
  turningPWM/1 -> Gain1/1
  Gain1/1 -> LCD1/1(In1)
  light/1 -> Gain/1
  Gain/1 -> LCD/1

== system et_robocon_dev_guy3/Main Controller/normal_operation_modes.see_saw/see_saw_mode.Speak ==
  f : TriggerPort  TriggerType=function-call
      settings: CopyFcn=Stateflow.SLINSF.SimulinkMan.removeBlockPreDeleteFcn  PreDeleteFcn=Stateflow.SLINSF.SimulinkMan.unsafePredeleteFcn
  Constant : Constant  Value=50
  Speaker : legonxtlib/Speaker  sinputMode=Volume only  sspeakerFreq=800  sspeakerVolume=50  sspeakerDuration=100
  wires:
  Constant/1 -> Speaker/1
